simulink model "Lab3Prob1"  (R2021a)
settings: Solver=VariableStepAuto  StartTime=0.0  StopTime=10.0  RelTol=1e-3
settings Model: Creator=emily  LastModifiedBy=emily

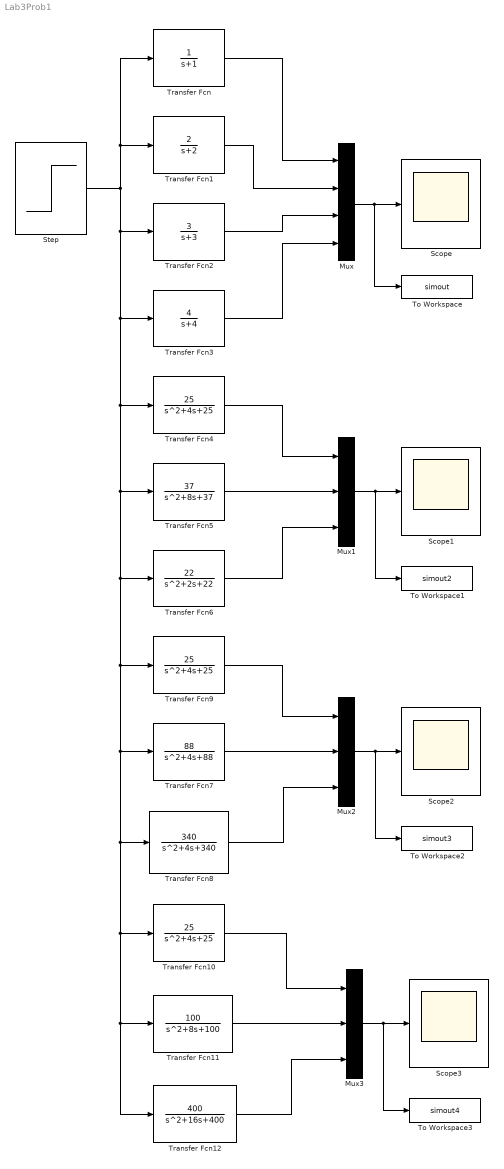
== system Lab3Prob1 ==
  Mux : Mux
  Mux1 : Mux  Inputs=3
  Mux2 : Mux  Inputs=3
  Mux3 : Mux  Inputs=3
  Scope{,1..3} (4 alike) : Scope
  Step : Step  SampleTime=0.01
  To Workspace : ToWorkspace  VariableName=simout  SaveFormat=Timeseries  SampleTime=-1
  To Workspace1 : ToWorkspace  VariableName=simout2  SaveFormat=Timeseries  SampleTime=-1
  To Workspace2 : ToWorkspace  VariableName=simout3  SaveFormat=Timeseries  SampleTime=-1
  To Workspace3 : ToWorkspace  VariableName=simout4  SaveFormat=Timeseries  SampleTime=-1
  Transfer Fcn : TransferFcn  Denominator=[1 1]
  Transfer Fcn1 : TransferFcn  Numerator=[2]  Denominator=[1 2]
  Transfer Fcn10 : TransferFcn  Numerator=[25]  Denominator=[1 4 25]
  Transfer Fcn11 : TransferFcn  Numerator=[100]  Denominator=[1 8 100]
  Transfer Fcn12 : TransferFcn  Numerator=[400]  Denominator=[1 16 400]
  Transfer Fcn2 : TransferFcn  Numerator=[3]  Denominator=[1 3]
  Transfer Fcn3 : TransferFcn  Numerator=[4]  Denominator=[1 4]
  Transfer Fcn4 : TransferFcn  Numerator=[25]  Denominator=[1 4 25]
  Transfer Fcn5 : TransferFcn  Numerator=[37]  Denominator=[1 8 37]
  Transfer Fcn6 : TransferFcn  Numerator=[22]  Denominator=[1 2 22]
  Transfer Fcn7 : TransferFcn  Numerator=[88]  Denominator=[1 4 88]
  Transfer Fcn8 : TransferFcn  Numerator=[340]  Denominator=[1 4 340]
  Transfer Fcn9 : TransferFcn  Numerator=[25]  Denominator=[1 4 25]
  wires:
  Step/1 -> Transfer Fcn1/1, Transfer Fcn/1, Transfer Fcn2/1, Transfer Fcn12/1, Transfer Fcn11/1, Transfer Fcn10/1, Transfer Fcn8/1, Transfer Fcn7/1, Transfer Fcn9/1, Transfer Fcn6/1, Transfer Fcn5/1, Transfer Fcn4/1, Transfer Fcn3/1
  Transfer Fcn/1 -> Mux/1
  Transfer Fcn1/1 -> Mux/2
  Transfer Fcn3/1 -> Mux/4
  Transfer Fcn2/1 -> Mux/3
  Mux/1 -> To Workspace/1, Scope/1
  Transfer Fcn5/1 -> Mux1/2
  Transfer Fcn4/1 -> Mux1/1
  Transfer Fcn6/1 -> Mux1/3
  Mux1/1 -> To Workspace1/1, Scope1/1
  Transfer Fcn9/1 -> Mux2/1
  Mux2/1 -> To Workspace2/1, Scope2/1
  Transfer Fcn7/1 -> Mux2/2
  Transfer Fcn8/1 -> Mux2/3
  Transfer Fcn12/1 -> Mux3/3
  Transfer Fcn11/1 -> Mux3/2
  Mux3/1 -> To Workspace3/1, Scope3/1
  Transfer Fcn10/1 -> Mux3/1
